simulink model "UNO_Traffic_light_task"  (Simulink 3.00)
libraries: logiclib x3, genlib x3, REXduino_library x2, mathlib x2, execlib x1

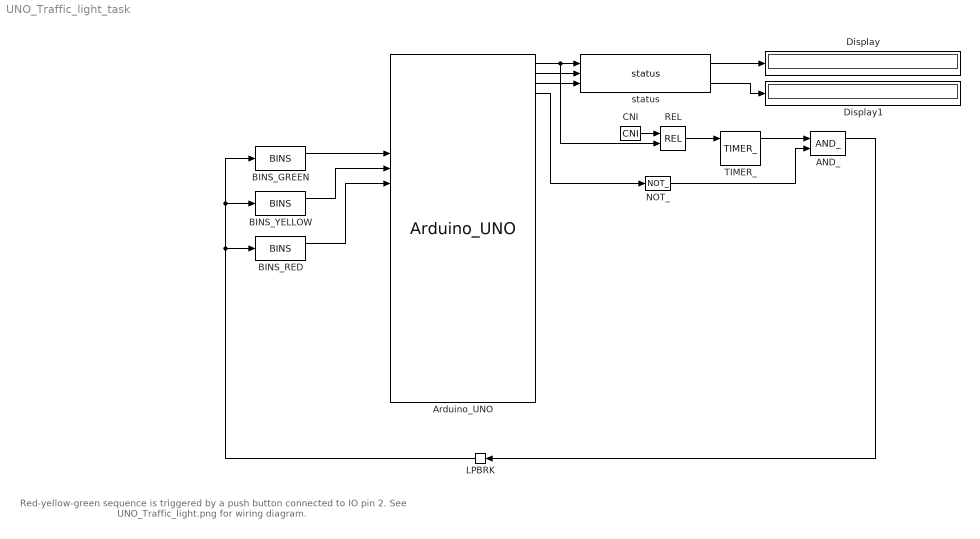
== system UNO_Traffic_light_task ==
  note: Red-yellow-green sequence is triggered by a push button connected to IO pin 2.
      |
      | See UNO_Traffic_light.png for wiring diagram.
  AND_ : logiclib/AND_
  Arduino_UNO : REXduino_library/Arduino_UNO  comPort=/dev/ttyACM0  pinmode2=4: Digital input with internal pull-up  pinmode3=1: Not connected  pinmode4=1: Not connected  pinmode5=1: Not connected  pinmode6=1: Not connected  pinmode9=2: Digital output  pinmode10=2: Digital output  pinmode11=2: Digital output  pinmodeA0=1: Not connected  pinmodeA1=1: Not connected  pinmodeA2=1: Not connected  pinmodeA3=1: Not connected  pinmodeA4=1: Not connected  pinmodeA5=1: Not connected  usercmd=1: No data
  BINS_GREEN : genlib/BINS  Y0=on  t1=0  t2=10  t3=0  t4=4  t5=5  t6=6  t7=7  t8=8  RPT=off
  BINS_RED : genlib/BINS  Y0=off  t1=2  t2=10  t3=0  t4=4  t5=5  t6=6  t7=7  t8=8  RPT=off
  BINS_YELLOW : genlib/BINS  Y0=off  t1=0  t2=2  t3=8  t4=10  t5=0  t6=6  t7=7  t8=8  RPT=off
  CNI : mathlib/CNI  icn=3
  Display : Display
      settings: Format=Best fit
  Display1 : Display
      settings: Format=Best fit
  LPBRK : execlib/LPBRK  Orientation=left
  NOT_ : logiclib/NOT_
  REL : mathlib/REL  irel=1: equality (==)
  TIMER_ : logiclib/TIMER_  mode=2: Delayed ON  pt=1
  status : REXduino_library/status
      mask Type: REX sequence
  wires:
  AND_/1 -> LPBRK/1
  Arduino_UNO/1 -> REL/2, status/1
  Arduino_UNO/2 -> status/2
  Arduino_UNO/3 -> status/3
  Arduino_UNO/4 -> NOT_/1
  BINS_GREEN/1 -> Arduino_UNO/6
  BINS_RED/1 -> Arduino_UNO/8
  BINS_YELLOW/1 -> Arduino_UNO/7
  CNI/1 -> REL/1
  LPBRK/1 -> BINS_RED/1, BINS_GREEN/1, BINS_YELLOW/1
  NOT_/1 -> AND_/2
  REL/1 -> TIMER_/1
  TIMER_/1 -> AND_/1
  status/1 -> Display/1
  status/2 -> Display1/1
